simulink model "FAN_FW"  (R2018b)
settings: Solver=ode45  StartTime=0.0  StopTime=40  FixedStep=Ts  RelTol=1e-4  EnableMultiTasking=on
InitFcn:
  | Ts = 1e-4;
  | 
  | Rs = 40;
  | Ld = 0.22;
  | Lq = 0.25;
  | Pn = 4;
  | flux = 0.195;
  | J = 0.000311;
  | 
  | umax = 311/sqrt(3);
  | 
  | kp_cur = Ld*1142;
  | ki_cur = Rs*1142;
  | 
  | 
  | kp_speed = 2*1.7*1*2*pi*J/2;
  | ki_speed = J*(1*2*pi/2)^2;
  | 
  | %kp_speed = 0.0195/5;
  | %ki_speed = 0.0195*50/25;
  | 
  | kp_comp = 0.65;
  | ki_comp = 0.001*pi*kp_comp;
  | 
  | %kp_FW = 0.004;
  | %ki_FW = 0.008;
  | 
  | kp_FW = 0.00004;
  | ki_FW = 0.0004;
  | %kp_FW = 0.00004;
  | %ki_FW = 0.0004;
undefined symbols (not defined in the file or in its folder): DiscIntNeverNeededParam
libraries: powerlib x5, simulink x4
Description:
  | %2020.11.18 98X机型
  | %Rs = 1.415;
  | %Ld = 15.05e-3;
  | %Lq = 18.65e-3;
  | %Pn = 3;
  | %flux = 0.222;
  | %J = 0.000355;
  | %kp_cur = Ld*590.7;
  | %ki_cur = Rs*590.7;
  | %kp_speed = 2*1.7*1*2*pi*J;
  | %ki_speed = J*(1*2*pi)^2;
  | %kp_FW = 0.0001;
  | %ki_FW = 0.00001;
  | 
  | %2020.11.18 海信机型
  | %Rs = 0.8975;
  | %Ld = 15e-3;
  | %Lq = 19e-3;
  | %Pn = 3;
  | %flux = 0.1764;
  | %J = 0.000311;
  | 
  | %2020.11.18 风机机型
  | %Rs = 49.5;
  | %Ld = 0.22;
  | %Lq = 0.25;
  | %Pn = 4;
  | %flux = 0.195;
  | %J = 0.000311;
settings Model: Creator=SUN  LastModifiedBy=liangjin
settings SolverCC: ZeroCrossControl=DisableAll
settings DataIOCC: LimitDataPoints=on  SaveFormat=Array
settings OptimizationCC: ExpressionDepthLimit=2147483647  InitFltsAndDblsToZero=on  LifeSpan=inf
settings DebuggingCC: UnderspecifiedInitializationDetection=Classic  MergeDetectMultiDrivingBlocksExec=none  SolverPrmCheckMsg=warning  FcnCallInpInsideContextMsg=warning  StateNameClashWarn=warning  SFUnexpectedBacktrackingDiag=warning  SFNoUnconditionalDefaultTransitionDiag=warning  SFExecutionAtInitializationDiag=none
settings HardwareCC: ProdBitPerPointer=32  ProdBitPerSizeT=32  ProdBitPerPtrDiffT=32  ProdLargestAtomicFloat=None  ProdIntDivRoundTo=Undefined  ProdEndianess=Unspecified  ProdWordSize=32  ProdHWDeviceType=32-bit Generic
settings ModelReferenceCC: PropagateSignalLabelsOutOfModel=off
settings SFSimCC: SimUseLocalCustomCode=off
settings RTWCC: RTWUseLocalCustomCode=off
settings CodeAppCC: StateflowObjectComments=on
settings GRTTargetCC: TargetLangStandard=C89/C90 (ANSI)  GeneratePreprocessorConditionals=Disable all  CombineOutputUpdateFcns=off  GRTInterface=on
settings ConfigComp: CovMetricSettings=dw  CovHtmlReporting=on  CovSaveCumulativeToWorkspaceVar=on  CovSaveSingleToWorkspaceVar=on  CovExternalEMLEnable=off  CovSFcnEnable=off
settings SimscapeCC: SimscapeNormalizeSystem=off

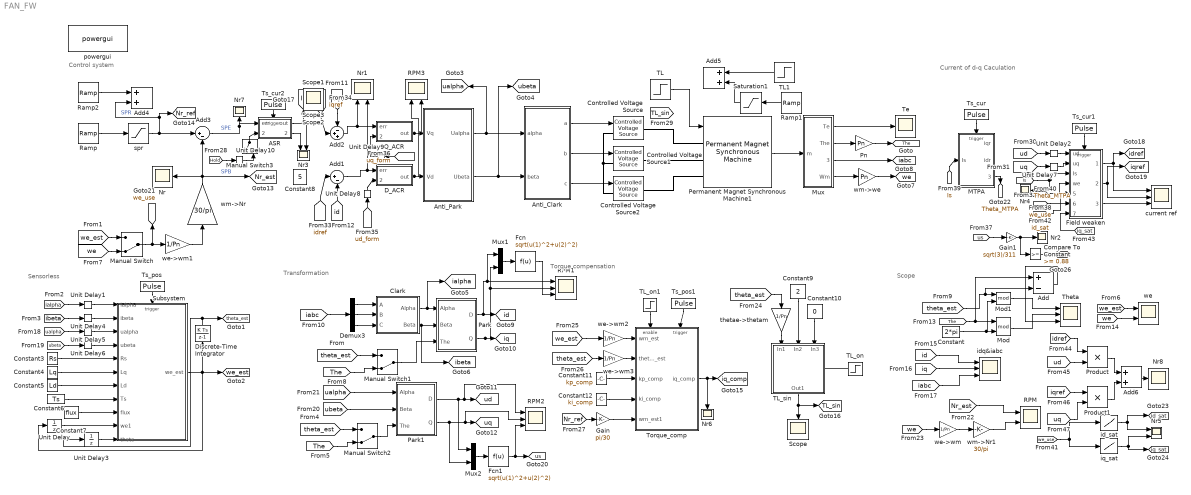
== system FAN_FW ==
  note: Torque compensation
  note: Scope
  note: Control system
  note: Transformation
  note: Sensorless
  note: Current of d-q Caculation
  ASR : Subsystem
  Add : Sum  Inputs=+-
  Add1 : Sum  Inputs=|+-
  Add2 : Sum  Inputs=-++
  Add3 : Sum  Inputs=|+-
  Add4 : Sum
  Add5 : Sum
  Add6 : Sum
  Anti_Clark : Subsystem
  Anti_Park : Subsystem
  Clark : Subsystem
  Compare To Constant : simulink/Logic and Bit Operations/Compare To Constant  relop=>=  const=0.88  OutDataTypeStr=boolean
  Constant : Constant  Value=2*pi
  Constant10 : Constant  Value=0
  Constant11 : Constant  Value=kp_comp
  Constant12 : Constant  Value=ki_comp
  Constant3 : Constant  Value=Rs
  Constant4 : Constant  Value=Lq
  Constant5 : Constant  Value=Ld
  Constant6 : Constant  Value=Ts
  Constant7 : Constant  Value=flux
  Constant8 : Constant  Value=5
  Constant9 : Constant  Value=2  SampleTime=Ts
  Controlled Voltage Source : powerlib/Electrical Sources/Controlled Voltage Source  Initialize=on  Source_Type=AC  Amplitude=0  Phase=0  Frequency=0  Measurements=Voltage
      settings: SourceProductName=Simscape Electrical
  Controlled Voltage Source1 : powerlib/Electrical Sources/Controlled Voltage Source  Initialize=on  Source_Type=AC  Amplitude=0  Phase=0  Frequency=0  Measurements=Voltage
      settings: SourceProductName=Simscape Electrical
  Controlled Voltage Source2 : powerlib/Electrical Sources/Controlled Voltage Source  Initialize=on  Source_Type=AC  Amplitude=0  Phase=0  Frequency=0  Measurements=Voltage
      settings: SourceProductName=Simscape Electrical
  D_ACR : Subsystem
  Demux3 : Demux  Outputs=3
  Discrete-Time Integrator : DiscreteIntegrator  gainval=1  SampleTime=Ts  ICPrevOutput=DiscIntNeverNeededParam  ICPrevScaledInput=DiscIntNeverNeededParam
  Fcn : Fcn  Expr=sqrt(u(1)^2+u(2)^2)
  Fcn1 : Fcn  Expr=sqrt(u(1)^2+u(2)^2)
  Field weaken : Subsystem
  Gain : Gain  Gain=pi/30
  Gain1 : Gain  Gain=sqrt(3)/311
  MTPA : Subsystem
  Manual Switch : ManualSwitch  CurrentSetting=0
  Manual Switch1 : ManualSwitch  CurrentSetting=0
  Manual Switch2 : ManualSwitch  CurrentSetting=0
  Manual Switch3 : ManualSwitch
  Mod : Math  Operator=mod  SaturateOnIntegerOverflow=on
  Mod1 : Math  Operator=mod  SaturateOnIntegerOverflow=on
  Mux : Subsystem
  Mux1 : Mux  Inputs=2
  Mux2 : Mux  Inputs=2
  Nr{,2,4,6..8} (6 alike) : Scope
  Nr1 : Scope  NumInputPorts=2
  Nr3 : Scope  NumInputPorts=2
  Nr5 : Scope  NumInputPorts=2
  Park : Subsystem
  Park1 : Subsystem
  Permanent Magnet Synchronous Machine1 : powerlib/Machines/Permanent Magnet Synchronous Machine  NbPhases=3  FluxDistribution=Sinusoidal  RotorType=Salient-pole  MechanicalLoad=Torque Tm  PresetModel=No  ShowDetailedParameters=on  MeasurementBus=off  Resistance=40  Inductance=8.5e-3  dqInductances=[0.22,0.25]  La=0.000835  MachineConstant=Flux linkage established by magnets (V.s)  Flux=0.195  VoltageCst=141.4764  TorqueCst=1.17  Flat=120  Mechanical=[0.000311 0.0000001 4 0]  PolePairs=3  InitialConditions=[0,0, 0,0]  InitialConditions5ph=[0 0 0 0 0 0]  TsPowergui=0  TsBlock=Ts  RefAngle=Aligned with phase A axis (original Park)
  Pn : Gain  Gain=Pn
  Product : Product
  Product1 : Product
  Q_ACR : Subsystem
  RPM : Scope  NumInputPorts=2
  RPM1 : Scope  NumInputPorts=3
  RPM2 : Scope  NumInputPorts=3
  RPM3 : Scope  NumInputPorts=2
  Ramp : simulink/Sources/Ramp  slope=500  start=0  InitialOutput=0
  Ramp1 : simulink/Sources/Ramp  slope=0.2  start=1  InitialOutput=0
  Ramp2 : simulink/Sources/Ramp  slope=-500  start=18  InitialOutput=0
  Saturation1 : Saturate  UpperLimit=4  LowerLimit=0
  Scope{,1..3} (4 alike) : Scope
  Subsystem : Subsystem
  TL : Step  After=0.8  SampleTime=Ts
  TL1 : Step  Time=15  After=-1  SampleTime=Ts
  TL_on : Step  Time=4  SampleTime=0
  TL_on1 : Step  Time=4  SampleTime=0
  TL_sin : Subsystem
  Te : Scope
  Theta : Scope  NumInputPorts=3
  Torque_comp : Subsystem
  Ts_cur : DiscretePulseGenerator  PulseType=Time based  Period=Ts  PulseWidth=50
  Ts_cur1 : DiscretePulseGenerator  PulseType=Time based  Period=Ts  PulseWidth=50
  Ts_cur2 : DiscretePulseGenerator  PulseType=Time based  Period=Ts  PulseWidth=50
  Ts_pos : DiscretePulseGenerator  PulseType=Time based  Period=Ts  PulseWidth=50
  Ts_pos1 : DiscretePulseGenerator  PulseType=Time based  Period=Ts  PulseWidth=50
  Unit Delay{,1..7} (8 alike) : UnitDelay  SampleTime=Ts
  Unit Delay10 : UnitDelay  SampleTime=-1
  Unit Delay8 : UnitDelay  SampleTime=-1
  Unit Delay9 : UnitDelay  SampleTime=-1
  current ref : Scope  NumInputPorts=3
  id_sat : Lookup_n-D  NumberOfTableDimensions=1  BreakpointsForDimension1=[20:20:4000]  Table=|  InternalRulePriority=Speed  RndMeth=Simplest  InputSameDT=on
      | [0
      | 0
      | 0
      | 0
      | 0
      | 0
      | 0
      | 0
      | 0
      | 0
      | 0
      | 0
      | 0
      | 0
      | 0
      | 0
      | 0
      | 0
      | 0
      | 0
      | 0
      | 0
      | 0
      | 0
      | 0
      | 0
      | 0
      | 0
      | 0
      | 0
      | 0
      | 0
      | 0
      | 0
      | -1.4282156
      | -1.993261291
      | -2.500274735
      | -2.95762852
      | -3.372109996
      | -3.749295371
      | -4.093818374
      | -4.409567747
      | -4.699835339
      | -4.967429105
      | -5.214760613
      | -5.443913731
      | -5.656699168
      | -5.854698247
      | -6.039298363
      | -6.211721953
      | -6.373050352
      | -6.524243572
      | -6.666156819
      | -6.799554349
      | -6.925121177
      | -7.043473009
      | -7.155164714
      | -7.260697576
      | -7.360525538
      | -7.455060585
      | -7.544677419
      | -7.629717516
      | -7.710492675
      | -7.78728811
      | -7.860365185
      | -7.9299638
      | -7.996304512
      | -8.059590407
      | -8.120008759
      | -8.177732505
      | -8.232921567
      | -8.285724019
      | -8.336277143
      | -8.38470837
      | -8.43113613
      | -8.475670606
      | -8.518414431
      | -8.559463299
      | -8.598906531
      | -8.636827584
      | -8.673304508
      | -8.708410367
      | -8.74221362
      | -8.774778469
      | -8.806165173
      | -8.836430342
      | -8.865627195
      | -8.89380581
      | -8.92101334
      | -8.947294219
      | -8.972690352
      | -8.997241281
      | -9.020984353
      | -9.043954856
      | -9.066186163
      | -9.087709851
      | -9.108555817
      | -9.128752388
      | -9.148326416
      | -9.167303371
      | -9.185707429
      | -9.203561544
      | -9.220887527
      | -9.237706113
      | -9.254037024
      | -9.269899028
      | -9.285309992
      | -9.30028694
      | -9.314846093
      | -9.329002919
      | -9.342772173
      | -9.356167938
      | -9.369203658
      | -9.381892176
      | -9.394245766
      | -9.406276161
      | -9.417994582
      | -9.429411766
      | -9.440537991
      | -9.451383096
      | -9.46195651
      | -9.472267265
      | -9.48232402
      | -9.492135081
      | -9.501708414
      | -9.511051664
      | -9.52017217
      | -9.52907698
      | -9.537772864
      | -9.546266329
      | -9.554563629
      | -9.562670776
      | -9.570593555
      | -9.57833753
      | -9.585908059
      | -9.593310297
      | -9.60054921
      | -9.607629581
      | -9.61455602
      | -9.621332968
      | -9.627964709
      | -9.634455372
      | -9.640808941
      | -9.64702926
      | -9.653120038
      | -9.659084857
      | -9.664927176
      | -9.670650332
      | -9.676257554
      | -9.681751959
      | -9.687136559
      | -9.692414269
      | -9.697587906
      | -9.702660194
      | -9.707633768
      | -9.71251118
      | -9.717294898
      | -9.721987311
      | -9.726590734
      | -9.731107406
      | -9.735539499
      | -9.739889116
      | -9.744158294
      | -9.748349008
      | -9.752463174
      | -9.756502648
      | -9.76046923
      | -9.764364667
      | -9.768190654
      | -9.771948834
      | -9.775640804
      | -9.779268112
      | -9.782832262
      | -9.786334715
      | -9.789776889
      | -9.793160162
      | -9.796485872
      | -9.799755319
      | -9.802969768
      | -9.806130448
      | -9.809238552
      | -9.812295243
      | -9.81530165
      | -9.818258872
      | -9.821167977
      | -9.824030004
      | -9.826845967
      | -9.82961685
      | -9.83234361
      | -9.835027183
      | -9.837668475
      | -9.840268372
      | -9.842827735
      | -9.845347404
      | -9.847828197
      | -9.850270911
      | -9.852676321
      | -9.855045185
      | -9.85737824
      | -9.859676205
      | ]
  idq&iabc : Scope  NumInputPorts=3
  iq_sat : Lookup_n-D  NumberOfTableDimensions=1  BreakpointsForDimension1=[20:20:4000]  Table=|  InternalRulePriority=Speed  RndMeth=Simplest  InputSameDT=on
      | [10
      | 10
      | 10
      | 10
      | 10
      | 10
      | 10
      | 10
      | 10
      | 10
      | 10
      | 10
      | 10
      | 10
      | 10
      | 10
      | 10
      | 10
      | 10
      | 10
      | 10
      | 10
      | 10
      | 10
      | 10
      | 10
      | 10
      | 10
      | 10
      | 10
      | 10
      | 10
      | 10
      | 10
      | 9.897484539
      | 9.799332091
      | 9.682387425
      | 9.552613964
      | 9.414290955
      | 9.270533114
      | 9.123631465
      | 8.97528341
      | 8.826751825
      | 8.678977364
      | 8.532659125
      | 8.388313495
      | 8.246317634
      | 8.10694199
      | 7.970374852
      | 7.836741056
      | 7.706116351
      | 7.578538501
      | 7.454015915
      | 7.332534395
      | 7.214062426
      | 7.098555344
      | 6.985958625
      | 6.87621049
      | 6.769243961
      | 6.664988498
      | 6.563371287
      | 6.464318264
      | 6.36775492
      | 6.273606928
      | 6.18180064
      | 6.092263465
      | 6.004924158
      | 5.919713039
      | 5.836562153
      | 5.755405379
      | 5.67617851
      | 5.598819294
      | 5.523267457
      | 5.449464703
      | 5.377354699
      | 5.306883056
      | 5.237997288
      | 5.170646772
      | 5.104782705
      | 5.040358051
      | 4.977327487
      | 4.915647352
      | 4.855275587
      | 4.796171685
      | 4.738296629
      | 4.681612844
      | 4.626084136
      | 4.571675646
      | 4.518353792
      | 4.466086223
      | 4.41484177
      | 4.364590396
      | 4.315303153
      | 4.266952139
      | 4.219510452
      | 4.172952153
      | 4.127252226
      | 4.082386538
      | 4.038331808
      | 3.995065568
      | 3.952566132
      | 3.910812564
      | 3.869784647
      | 3.829462856
      | 3.789828327
      | 3.750862836
      | 3.712548767
      | 3.674869091
      | 3.637807343
      | 3.6013476
      | 3.565474459
      | 3.530173016
      | 3.495428846
      | 3.461227989
      | 3.427556926
      | 3.394402566
      | 3.36175223
      | 3.329593631
      | 3.297914864
      | 3.266704389
      | 3.23595102
      | 3.205643908
      | 3.175772532
      | 3.146326683
      | 3.117296459
      | 3.088672246
      | 3.060444715
      | 3.032604806
      | 3.005143721
      | 2.978052915
      | 2.951324087
      | 2.924949168
      | 2.898920319
      | 2.873229917
      | 2.847870553
      | 2.822835019
      | 2.798116307
      | 2.773707596
      | 2.749602251
      | 2.725793813
      | 2.702275997
      | 2.679042682
      | 2.656087907
      | 2.633405868
      | 2.61099091
      | 2.588837522
      | 2.566940337
      | 2.545294119
      | 2.523893767
      | 2.502734308
      | 2.481810888
      | 2.461118776
      | 2.440653356
      | 2.420410124
      | 2.400384682
      | 2.380572741
      | 2.360970112
      | 2.341572703
      | 2.32237652
      | 2.303377661
      | 2.284572314
      | 2.265956753
      | 2.24752734
      | 2.229280514
      | 2.211212798
      | 2.193320789
      | 2.175601161
      | 2.158050659
      | 2.1406661
      | 2.123444368
      | 2.106382414
      | 2.089477254
      | 2.072725965
      | 2.056125686
      | 2.039673615
      | 2.023367006
      | 2.00720317
      | 1.991179471
      | 1.975293326
      | 1.959542202
      | 1.943923615
      | 1.928435132
      | 1.913074362
      | 1.897838962
      | 1.882726634
      | 1.867735119
      | 1.852862202
      | 1.838105707
      | 1.823463498
      | 1.808933475
      | 1.794513578
      | 1.780201779
      | 1.765996087
      | 1.751894542
      | 1.73789522
      | 1.723996225
      | 1.710195695
      | 1.696491794
      | 1.682882717
      | 1.669366687
      | ]
  powergui : powerlib/powergui  SimulationMode=Discrete  SampleTime=1e-5  frequency=60  Iterations=50  frequencyindice=0  Pbase=100e6  ErrMax=1e-4  UnitsV=kV  UnitsW=MW  buscounter=0  FunctionMessages=off  echomessages=off  EnableUseOfTLC=off  CurrentSourceSwitches=off  DisableSnubberDevices=off  DisableRonSwitches=off  DisableVfSwitches=off  DisplayEquations=off  SolverType=Tustin/Backward Euler (TBE)  Interpol=off  ExternalGateDelay=off  methode=off  Ts=100  x0status=blocks  SPID=off  SwTol=0  HookPort=off  RestoreLinks=warning  ResistiveCurrentMeasurement=off  Frange=[0:2:500]  Ylog=off  Xlog=on  ShowGrid=off  save=off  variable=ZData  structure=0  ZoomFFT=on  StartTime=0.0  cycles=1  DisplayStyle=1  fundamental=60  FreqAxis=off  MaxFrequency=1000  frequencyindicesteady=1  RmsSteady=1  display=off
  spr : Saturate  UpperLimit=8000  LowerLimit=-1000
  thetae->thetam : Gain  Gain=1/Pn
  we : Scope  NumInputPorts=2
  we->wm{,1..3} (4 alike) : Gain  Gain=1/Pn
  wm->Nr : Gain  Gain=30/pi
  wm->Nr1 : Gain  Gain=30/pi
  wm->we : Gain  Gain=Pn
  tag scope: Hold=global, Is=global, Nr_est=global, Nr_ref=global, TL_sin=global, The=global, Theta_MTPA=global, iabc=global, ialpha=global, ibeta=global, id=global, id_sat=global, idref=global, iq=global, iq_comp=global, iq_sat=global, iqref=global, theta_est=global, ualpha=global, ubeta=global, ud=global, uq=global, us=global, we=global, we_est=global, we_use=global
  wires:
  Permanent Magnet Synchronous Machine1/1 -> Mux/1(m)
  Add3/1 -> ASR/1(err), Nr7/1  "SPE"
  wm->Nr/1 -> [Nr_est], Add3/2, Nr/1  "SPB"
  Mux/1(Te) -> Te/1
  Mux/2(The) -> Pn/1
  Pn/1 -> [The]
  Mux/4(Wm) -> wm->we/1
  Mux/3(Iabc) -> [iabc]
  Clark/1(Alpha) -> [ialpha], Park/1(Alpha)
  Demux3/1 -> Clark/1(A)
  Demux3/2 -> Clark/2(B)
  Demux3/3 -> Clark/3(C)
  Clark/2(Beta) -> Park/2(Beta), [ibeta]
  Q_ACR/1(out) -> RPM3/2, Anti_Park/1(Vq)
  D_ACR/1(out) -> RPM3/1, Anti_Park/2(Vd)
  Anti_Clark/2(b) -> Controlled Voltage Source1/1
  Anti_Clark/3(c) -> Controlled Voltage Source2/1
  Constant/1 -> Mod1/2, Mod/2
  Mod/1 -> Theta/2
  wm->we/1 -> [we]
  Ramp/1 -> spr/1
  we->wm1/1 -> wm->Nr/1
  [we_est] -> we/1
  [we_est] -> Manual Switch/1
  [we] -> Manual Switch/2
  [theta_est] -> Manual Switch1/1
  Manual Switch1/1 -> Park/3(The)
  [The] -> Manual Switch1/2
  Park/1(D) -> Mux1/1, RPM1/1, [id]
  Park/2(Q) -> Mux1/2, RPM1/2, [iq]
  [The] -> Add/1, Mod/1
  [id] -> idq&iabc/1
  [iq] -> idq&iabc/2
  [iabc] -> idq&iabc/3
  [id] -> Add1/2
  [iq] -> Add2/1
  Manual Switch/1 -> we->wm1/1, [we_use]
  [The] -> Manual Switch2/2
  Manual Switch2/1 -> Park1/3(The)
  [theta_est] -> Manual Switch2/1
  [ubeta] -> Park1/2(Beta)
  [ualpha] -> Park1/1(Alpha)
  Park1/1(D) -> Mux2/1, [ud], RPM2/1
  Park1/2(Q) -> Mux2/2, RPM2/2, [uq]
  Anti_Park/1(Ualpha) -> [ualpha], Anti_Clark/1(alpha)
  Anti_Park/2(Ubeta) -> [ubeta], Anti_Clark/2(beta)
  Subsystem/1(we_est) -> Discrete-Time Integrator/1, [we_est], Unit Delay/1
  Constant3/1 -> Subsystem/5(Rs)
  Constant4/1 -> Subsystem/6(Lq)
  Constant5/1 -> Subsystem/7(Ld)
  Constant6/1 -> Subsystem/8(Ts)
  Constant7/1 -> Subsystem/9(flux)
  Unit Delay/1 -> Subsystem/10(we1)
  Ts_pos/1 -> Subsystem/Trigger
  Unit Delay3/1 -> Subsystem/11(theta)
  [theta_est] -> Add/2, Mod1/1
  Mod1/1 -> Theta/1
  [iabc] -> Demux3/1
  Discrete-Time Integrator/1 -> [theta_est], Unit Delay3/1
  Anti_Clark/1(a) -> Controlled Voltage Source/1
  [ialpha] -> Unit Delay1/1
  [ibeta] -> Unit Delay4/1
  [ualpha] -> Unit Delay5/1
  [ubeta] -> Unit Delay6/1
  [we] -> we->wm/1
  we->wm/1 -> wm->Nr1/1
  wm->Nr1/1 -> RPM/2
  [Nr_est] -> RPM/1
  spr/1 -> [Nr_ref], Add4/2, Add3/1  "SPR"
  Ts_cur/1 -> MTPA/Trigger
  [we] -> we/2
  [theta_est] -> thetae->thetam/1
  thetae->thetam/1 -> TL_sin/1(In1)
  Constant9/1 -> TL_sin/2(In2)
  Constant10/1 -> TL_sin/3(In3)
  TL_on/1 -> TL_sin/Enable
  TL_sin/1(Out1) -> [TL_sin], Scope/1
  we->wm2/1 -> Torque_comp/1(wm_est)
  we->wm3/1 -> Torque_comp/2(thetam_est)
  Constant11/1 -> Torque_comp/3(kp_comp)
  Constant12/1 -> Torque_comp/4(ki_comp)
  Torque_comp/1(iq_comp) -> Nr6/1, [iq_comp]
  [Nr_ref] -> Gain/1
  Gain/1 -> Torque_comp/5(wm_est1)
  Ts_pos1/1 -> Torque_comp/Trigger
  TL_on1/1 -> Torque_comp/Enable
  [we_est] -> we->wm2/1
  [theta_est] -> we->wm3/1
  [ud] -> Unit Delay2/1
  [uq] -> Unit Delay7/1
  [Is] -> Nr4/1, Field weaken/3(Is)
  Ts_cur1/1 -> Field weaken/Trigger
  Field weaken/1(idref) -> current ref/1, [idref]
  Field weaken/2(iqref) -> [iqref], current ref/2
  Add/1 -> Theta/3
  Mux1/1 -> Fcn/1
  Field weaken/3(jiaodu) -> current ref/3
  Mux2/1 -> Fcn1/1
  Fcn1/1 -> [us], RPM2/3
  Unit Delay1/1 -> Subsystem/1(ialpha)
  Unit Delay4/1 -> Subsystem/2(ibeta)
  Unit Delay5/1 -> Subsystem/3(ualpha)
  Unit Delay6/1 -> Subsystem/4(ubeta)
  Unit Delay2/1 -> Field weaken/1(ud)
  Unit Delay7/1 -> Field weaken/2(uq)
  [ud_form] -> Unit Delay8/1
  Unit Delay8/1 -> D_ACR/2(ud_form)
  [uq_form] -> Unit Delay9/1
  Unit Delay9/1 -> Q_ACR/2(uq_form)
  [us] -> Gain1/1
  Gain1/1 -> Compare To Constant/1, Nr2/1
  [we_use] -> Field weaken/4(we)
  Ramp1/1 -> Saturation1/1
  Ramp2/1 -> Add4/1
  TL1/1 -> Add5/1
  [Is] -> MTPA/1(Is)
  MTPA/3(Theta_MTPA) -> [Theta_MTPA]
  [Theta_MTPA] -> Field weaken/5(Theta_MTPA)
  [we_use] -> id_sat/1, iq_sat/1
  id_sat/1 -> Nr5/1, [id_sat]
  iq_sat/1 -> [iq_sat], Nr5/2
  [id_sat] -> Field weaken/6(id_sat)
  [iq_sat] -> Field weaken/7(iq_sat)
  Add1/1 -> Nr1/2, D_ACR/1(err)
  Add2/1 -> Nr1/1, Q_ACR/1(err)
  ASR/1(out) -> Nr3/2, [Is]
  ASR/2(speed_sat) -> Nr3/1
  Compare To Constant/1 -> [Hold]
  [Hold] -> Unit Delay10/1
  Manual Switch3/1 -> ASR/2(Hold)
  Unit Delay10/1 -> Manual Switch3/2
  [idref] -> Product/1
  [ud] -> Product/2
  [iqref] -> Product1/1
  [uq] -> Product1/2
  Product/1 -> Add6/1
  Product1/1 -> Add6/2
  Add6/1 -> Nr8/1
  [idref] -> Add1/1
  [iqref] -> Add2/2
  Ts_cur2/1 -> ASR/Trigger
  Fcn/1 -> RPM1/3
  Saturation1/1 -> Add5/2
  TL/1 -> Permanent Magnet Synchronous Machine1/1
  connections:
  Controlled Voltage Source/LConn1 -- Controlled Voltage Source2/LConn1 -- Controlled Voltage Source1/LConn1
  Controlled Voltage Source/RConn1 -- Permanent Magnet Synchronous Machine1/LConn1
  Controlled Voltage Source1/RConn1 -- Permanent Magnet Synchronous Machine1/LConn2
  Controlled Voltage Source2/RConn1 -- Permanent Magnet Synchronous Machine1/LConn3

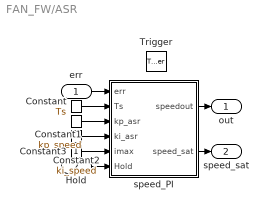
== system FAN_FW/ASR ==
  err : Inport
  Hold : Inport  Port=2
  Trigger : TriggerPort  VariantControl=Variant  PortDimensions=1
  Constant : Constant  Value=Ts
  Constant1 : Constant  Value=kp_speed
  Constant2 : Constant  Value=ki_speed
  Constant3 : Constant
  speed_PI : MATLAB Function  TreatAsAtomicUnit=on
  out : Outport
  speed_sat : Outport  Port=2
  wires:
  speed_PI/1(speedout) -> out/1
  speed_PI/2(speed_sat) -> speed_sat/1
  Hold/1 -> speed_PI/6(Hold)
  Constant2/1 -> speed_PI/4(ki_asr)
  Constant3/1 -> speed_PI/5(imax)
  Constant/1 -> speed_PI/2(Ts)
  err/1 -> speed_PI/1(err)
  Constant1/1 -> speed_PI/3(kp_asr)

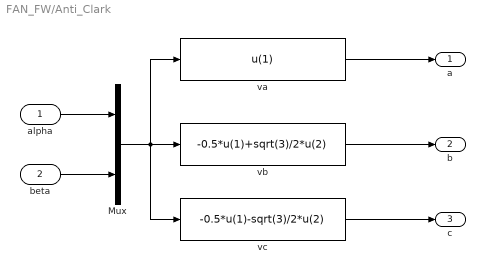
== system FAN_FW/Anti_Clark ==
  alpha : Inport
  beta : Inport  Port=2
  Mux : Mux  Inputs=2
  va : Fcn  Expr=u(1)
  vb : Fcn  Expr=-0.5*u(1)+sqrt(3)/2*u(2)
  vc : Fcn  Expr=-0.5*u(1)-sqrt(3)/2*u(2)
  a : Outport
  b : Outport  Port=2
  c : Outport  Port=3
  wires:
  va/1 -> a/1
  beta/1 -> Mux/2
  alpha/1 -> Mux/1
  Mux/1 -> vc/1, vb/1, va/1
  vb/1 -> b/1
  vc/1 -> c/1

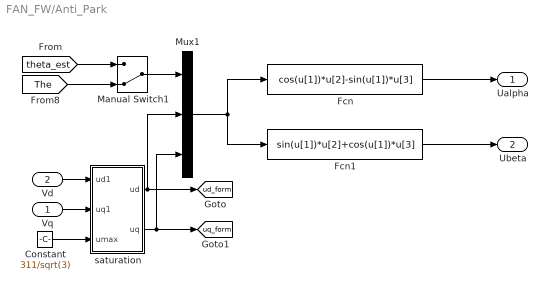
== system FAN_FW/Anti_Park ==
  Vq : Inport
  Vd : Inport  Port=2
  Constant : Constant  Value=311/sqrt(3)
  Fcn : Fcn  Expr=cos(u[1])*u[2]-sin(u[1])*u[3]
  Fcn1 : Fcn  Expr=sin(u[1])*u[2]+cos(u[1])*u[3]
  Manual Switch1 : ManualSwitch  CurrentSetting=0
  Mux1 : Mux  Inputs=3
  saturation : MATLAB Function  TreatAsAtomicUnit=on
  Ualpha : Outport
  Ubeta : Outport  Port=2
  tag scope: ud_form=global, uq_form=global
  wires:
  Fcn1/1 -> Ubeta/1
  Fcn/1 -> Ualpha/1
  Mux1/1 -> Fcn/1, Fcn1/1
  Manual Switch1/1 -> Mux1/1
  [The] -> Manual Switch1/2
  [theta_est] -> Manual Switch1/1
  Vd/1 -> saturation/1(ud1)
  Vq/1 -> saturation/2(uq1)
  saturation/1(ud) -> Mux1/2, [ud_form]
  saturation/2(uq) -> [uq_form], Mux1/3
  Constant/1 -> saturation/3(umax)

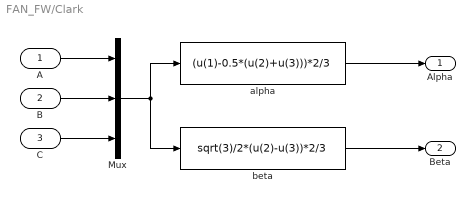
== system FAN_FW/Clark ==
  A : Inport
  B : Inport  Port=2
  C : Inport  Port=3
  Mux : Mux  Inputs=3
  alpha : Fcn  Expr=(u(1)-0.5*(u(2)+u(3)))*2/3
  beta : Fcn  Expr=sqrt(3)/2*(u(2)-u(3))*2/3
  Alpha : Outport
  Beta : Outport  Port=2
  wires:
  alpha/1 -> Alpha/1
  B/1 -> Mux/2
  C/1 -> Mux/3
  A/1 -> Mux/1
  Mux/1 -> beta/1, alpha/1
  beta/1 -> Beta/1

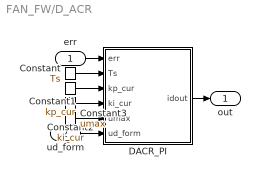
== system FAN_FW/D_ACR ==
  err : Inport
  ud_form : Inport  Port=2
  Constant : Constant  Value=Ts
  Constant1 : Constant  Value=kp_cur
  Constant2 : Constant  Value=ki_cur
  Constant3 : Constant  Value=umax
  DACR_PI : MATLAB Function  TreatAsAtomicUnit=on
  out : Outport
  wires:
  err/1 -> DACR_PI/1(err)
  Constant3/1 -> DACR_PI/5(umax)
  Constant2/1 -> DACR_PI/4(ki_cur)
  Constant/1 -> DACR_PI/2(Ts)
  Constant1/1 -> DACR_PI/3(kp_cur)
  ud_form/1 -> DACR_PI/6(ud_form)
  DACR_PI/1(idout) -> out/1

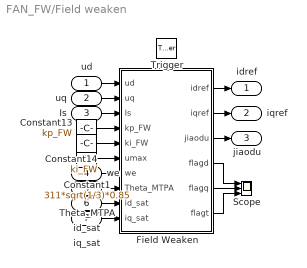
== system FAN_FW/Field weaken ==
  ud : Inport
  uq : Inport  Port=2
  Is : Inport  Port=3
  we : Inport  Port=4
  Theta_MTPA : Inport  Port=5
  id_sat : Inport  Port=6
  iq_sat : Inport  Port=7
  Trigger : TriggerPort  VariantControl=Variant  PortDimensions=1
  Constant1 : Constant  Value=311*sqrt(1/3)*0.85
  Constant13 : Constant  Value=kp_FW
  Constant14 : Constant  Value=ki_FW
  Field Weaken : MATLAB Function  TreatAsAtomicUnit=on
  Scope : Scope  NumInputPorts=3
  idref : Outport
  iqref : Outport  Port=2
  jiaodu : Outport  Port=3
  wires:
  Constant13/1 -> Field Weaken/4(kp_FW)
  Field Weaken/1(idref) -> idref/1
  Constant14/1 -> Field Weaken/5(ki_FW)
  uq/1 -> Field Weaken/2(uq)
  Constant1/1 -> Field Weaken/6(umax)
  Field Weaken/2(iqref) -> iqref/1
  ud/1 -> Field Weaken/1(ud)
  Is/1 -> Field Weaken/3(Is)
  Field Weaken/3(jiaodu) -> jiaodu/1
  we/1 -> Field Weaken/7(we)
  Theta_MTPA/1 -> Field Weaken/8(Theta_MTPA)
  Field Weaken/4(flagd) -> Scope/1
  Field Weaken/5(flagq) -> Scope/2
  Field Weaken/6(flagt) -> Scope/3
  id_sat/1 -> Field Weaken/9(id_sat)
  iq_sat/1 -> Field Weaken/10(iq_sat)

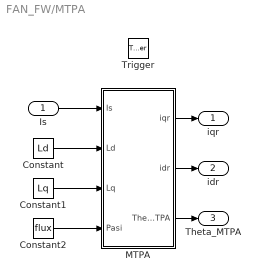
== system FAN_FW/MTPA ==
  Is : Inport
  Trigger : TriggerPort  VariantControl=Variant  PortDimensions=1
  Constant : Constant  Value=Ld
  Constant1 : Constant  Value=Lq
  Constant2 : Constant  Value=flux
  MTPA : MATLAB Function  TreatAsAtomicUnit=on
  iqr : Outport
  idr : Outport  Port=2
  Theta_MTPA : Outport  Port=3
  wires:
  MTPA/1(iqr) -> iqr/1
  Is/1 -> MTPA/1(Is)
  Constant/1 -> MTPA/2(Ld)
  Constant1/1 -> MTPA/3(Lq)
  Constant2/1 -> MTPA/4(Pasi)
  MTPA/2(idr) -> idr/1
  MTPA/3(Theta_MTPA) -> Theta_MTPA/1

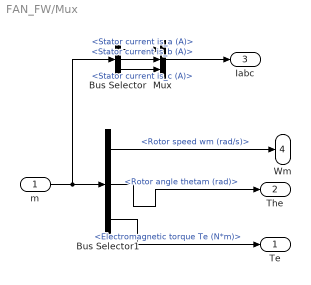
== system FAN_FW/Mux ==
  m : Inport
  Bus Selector : BusSelector  OutputSignals=Stator current is_a (A),Stator current is_b (A),Stator current is_c (A)
  Bus Selector1 : BusSelector  OutputSignals=Rotor speed wm (rad/s),Rotor angle thetam (rad),Electromagnetic torque Te (N*m)
  Mux : Mux  Inputs=3
  Te : Outport
  The : Outport  Port=2
  Iabc : Outport  Port=3
  Wm : Outport  Port=4
  wires:
  Bus Selector1/1 -> Wm/1  "<Rotor speed wm (rad/s)>"
  Bus Selector1/2 -> The/1  "<Rotor angle thetam (rad)>"
  Bus Selector1/3 -> Te/1  "<Electromagnetic torque Te (N*m)>"
  m/1 -> Bus Selector/1, Bus Selector1/1
  Bus Selector/2 -> Mux/2  "<Stator current is_b (A)>"
  Bus Selector/3 -> Mux/3  "<Stator current is_c (A)>"
  Bus Selector/1 -> Mux/1  "<Stator current is_a (A)>"
  Mux/1 -> Iabc/1

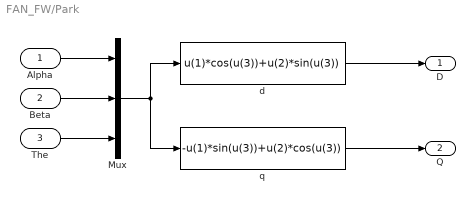
== system FAN_FW/Park ==
  Alpha : Inport
  Beta : Inport  Port=2
  The : Inport  Port=3
  Mux : Mux  Inputs=3
  d : Fcn  Expr=u(1)*cos(u(3))+u(2)*sin(u(3))
  q : Fcn  Expr=-u(1)*sin(u(3))+u(2)*cos(u(3))
  D : Outport
  Q : Outport  Port=2
  wires:
  d/1 -> D/1
  Beta/1 -> Mux/2
  Alpha/1 -> Mux/1
  Mux/1 -> q/1, d/1
  q/1 -> Q/1
  The/1 -> Mux/3

== system FAN_FW/Park1 ==
  Alpha : Inport
  Beta : Inport  Port=2
  The : Inport  Port=3
  Mux : Mux  Inputs=3
  d : Fcn  Expr=u(1)*cos(u(3))+u(2)*sin(u(3))
  q : Fcn  Expr=-u(1)*sin(u(3))+u(2)*cos(u(3))
  D : Outport
  Q : Outport  Port=2
  wires:
  d/1 -> D/1
  Beta/1 -> Mux/2
  Alpha/1 -> Mux/1
  Mux/1 -> q/1, d/1
  q/1 -> Q/1
  The/1 -> Mux/3

== system FAN_FW/Q_ACR ==
  err : Inport
  uq_form : Inport  Port=2
  Constant : Constant  Value=Ts
  Constant1 : Constant  Value=kp_cur
  Constant2 : Constant  Value=ki_cur
  Constant3 : Constant  Value=umax
  QACR_PI : MATLAB Function  TreatAsAtomicUnit=on
  out : Outport
  wires:
  err/1 -> QACR_PI/1(err)
  Constant3/1 -> QACR_PI/5(umax)
  Constant2/1 -> QACR_PI/4(ki_cur)
  Constant/1 -> QACR_PI/2(Ts)
  Constant1/1 -> QACR_PI/3(kp_cur)
  uq_form/1 -> QACR_PI/6(ud_form)
  QACR_PI/1(iqout) -> out/1

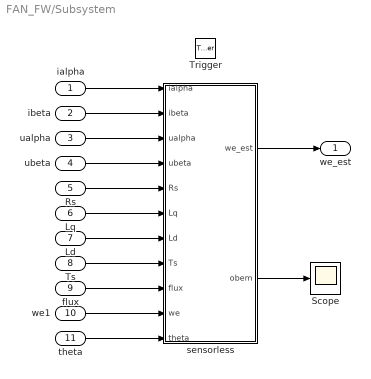
== system FAN_FW/Subsystem ==
  ialpha : Inport
  ibeta : Inport  Port=2
  ualpha : Inport  Port=3
  ubeta : Inport  Port=4
  Rs : Inport  Port=5
  Lq : Inport  Port=6
  Ld : Inport  Port=7
  Ts : Inport  Port=8
  flux : Inport  Port=9
  we1 : Inport  Port=10
  theta : Inport  Port=11
  Trigger : TriggerPort  VariantControl=Variant  PortDimensions=1
  Scope : Scope
  sensorless : MATLAB Function  TreatAsAtomicUnit=on
  we_est : Outport
  wires:
  ualpha/1 -> sensorless/3(ualpha)
  Ts/1 -> sensorless/8(Ts)
  flux/1 -> sensorless/9(flux)
  ialpha/1 -> sensorless/1(ialpha)
  sensorless/1(we_est) -> we_est/1
  Lq/1 -> sensorless/6(Lq)
  ubeta/1 -> sensorless/4(ubeta)
  ibeta/1 -> sensorless/2(ibeta)
  Rs/1 -> sensorless/5(Rs)
  Ld/1 -> sensorless/7(Ld)
  we1/1 -> sensorless/10(we)
  theta/1 -> sensorless/11(theta)
  sensorless/2(obem) -> Scope/1

== system FAN_FW/TL_sin ==
  In1 : Inport
  In2 : Inport  Port=2
  In3 : Inport  Port=3
  Enable : EnablePort
  MATLAB Function : MATLAB Function  TreatAsAtomicUnit=on
  Out1 : Outport
  wires:
  In1/1 -> MATLAB Function/1(Theta_m)
  MATLAB Function/1(TL) -> Out1/1
  In3/1 -> MATLAB Function/3(Theta0)
  In2/1 -> MATLAB Function/2(Amp)

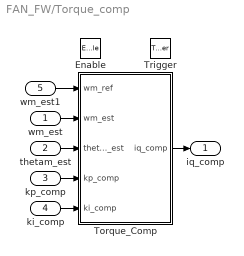
== system FAN_FW/Torque_comp ==
  wm_est : Inport
  thetam_est : Inport  Port=2
  kp_comp : Inport  Port=3
  ki_comp : Inport  Port=4
  wm_est1 : Inport  Port=5
  Enable : EnablePort
  Trigger : TriggerPort  VariantControl=Variant  PortDimensions=1
  Torque_Comp : MATLAB Function  TreatAsAtomicUnit=on
  iq_comp : Outport
  wires:
  Torque_Comp/1(iq_comp) -> iq_comp/1
  kp_comp/1 -> Torque_Comp/4(kp_comp)
  wm_est/1 -> Torque_Comp/2(wm_est)
  ki_comp/1 -> Torque_Comp/5(ki_comp)
  wm_est1/1 -> Torque_Comp/1(wm_ref)
  thetam_est/1 -> Torque_Comp/3(thetam_est)

== matlab function FAN_FW/MTPA/MTPA ==
  data: iqr output; Is input; idr output; Ld input; Lq input; Pasi input; Theta_MTPA output
function [iqr,idr,Theta_MTPA] = MTPA(Is,Ld,Lq,Pasi)

persistent id1 iq1;

if isempty(id1)
    id1=0;iq1=0;
end

iq1 = Is;
id1 = iq1*iq1*(Ld-Lq)/Pasi;

Theta_MTPA = atan(id1/iq1);
idr = id1;
iqr = iq1;

== matlab function FAN_FW/Subsystem/sensorless ==
  data: ialpha input; we_est output; ibeta input; ualpha input; ubeta input; Rs input; Lq input; Ld input; Ts input; flux input; we input; theta input; obem output

function [we_est, obem]  = sensorless(ialpha,ibeta,ualpha,ubeta,Rs,Lq,Ld,Ts,flux,we,theta)

persistent id2 iq2 delta_id delta_iq bemf we1 flag;

if isempty(id2)
    id2=0;iq2=0;delta_id=0;delta_iq=0;bemf=0;we1=0;flag=0;obem=0;
end

ud= cos(theta)*ualpha+sin(theta)*ubeta;
uq=-sin(theta)*ualpha+cos(theta)*ubeta;
id1= cos(theta)*ialpha+sin(theta)*ibeta;
iq1=-sin(theta)*ialpha+cos(theta)*ibeta;

if(bemf < 0)
    flag = 1;
end

we1 = we1+0.715*(we-we1);
temp1 = ud-id2*Rs;
temp1 = temp1+we1*Lq*iq2;
temp1 = temp1*Ts/Ld + id2;
delta_id = delta_id+0.125*((temp1-id1)-delta_id);

temp2 = uq-iq2*Rs;
temp2 = temp2-we1*Ld*id2;
temp2 = temp2-bemf;
temp2 = Ts*temp2/Lq+iq2;
delta_iq = delta_iq+0.5*((temp2-iq1)-delta_iq);

bemf = bemf+delta_iq*Lq/Ts;
if(flag)
    we_est = (bemf+delta_id*Ld/Ts)/flux;
else
    we_est = (bemf-delta_id*Ld/Ts)/flux;
end

obem = bemf;
id2 = id1;
iq2 = iq1;

== matlab function FAN_FW/TL_sin/MATLAB Function ==
  data: Theta_m input; TL output; Amp input; Theta0 input
function TL = fcn(Theta_m,Amp,Theta0)
if isempty(Theta_m)
    Theta_m=0;Amp=0;Theta0=0;TL=0;
end
TL = Amp*sin(Theta_m+Theta0);

== matlab function FAN_FW/Torque_comp/Torque_Comp ==
  data: wm_ref input; iq_comp output; wm_est input; thetam_est input; kp_comp input; ki_comp input
function iq_comp = Torque_Comp(wm_ref,wm_est,thetam_est,kp_comp,ki_comp)

persistent Te temp1 temp2 up ui1 ui2 out1 out2 comp1_fbk comp2_fbk comp1_ref comp2_ref;

if isempty(temp1)
    Te=0; temp1=0; temp2=0; up=0; ui1=0; ui2=0; out1=0; out2=0; iq_comp=0; 
    comp1_fbk=0; comp2_fbk=0; comp1_ref=0; comp2_ref=0;
end

%calc comp sin value
Te = wm_ref-wm_est;
temp1 = Te*sin(thetam_est);
comp1_fbk = 0;
if (wm_ref < 10)
    comp1_ref = 0;
else
    comp1_ref = temp1;
end
up = comp1_ref - comp1_fbk;
ui1 = ui1 + ki_comp*up;
out1 = kp_comp*up + ui1;

%calc comp cos value
temp2 = Te*cos(thetam_est);
comp2_fbk = 0;
if (wm_ref < 10)
    comp2_ref = 0;
else
    comp2_ref = temp2;
end
up = comp2_ref - comp2_fbk;
ui2 = ui2 + ki_comp*up;
out2 = kp_comp*up + ui2;

iq_comp = out1*sin(thetam_est) + out2*cos(thetam_est);

if (iq_comp > 10)
    iq_comp = 10;
elseif (iq_comp < -10)
    iq_comp = -10;
end

== matlab function FAN_FW/Field weaken/Field Weaken ==
  data: idref output; iqref output; ud input; uq input; Is input; kp_FW input; ki_FW input; umax input; jiaodu output; we input; Theta_MTPA input; flagd output; flagq output; flagt output; id_sat input; iq_sat input
function [idref,iqref,jiaodu,flagd,flagq,flagt] = Fieldweaken(ud,uq,Is,kp_FW,ki_FW,umax,we,Theta_MTPA,id_sat,iq_sat)

persistent us gama uout ui temp id1 iq1 gama_sat upper flag_temp1 flag_temp2 flag_temp3 ;

if isempty(us)
    us=0;gama=0;ui=0;temp=0;uout=0;id1=0;iq1=0;gama_sat=0;upper=0;flag_temp1=0;flag_temp2=0;flag_temp3=0;
%     id_sat=0;iq_sat=0;
end
% 
% id_sat = (5.385-0.01537*we+0.000004*we*we);
% iq_sat = (16.82-0.01108*we+0.000002*we*we);
% id_sat = (9.3451-0.0243*we+0.00001*we*we-2*10^(-9)*we*we*we);
% iq_sat = (15.36-0.0085*we+0.000002*we*we);


%gama_sat = k1*asin(id_sat/10);

flag_temp2 = 0;
flag_temp3 = 0;
us = sqrt(ud.^2+uq.^2);
temp = umax - us;

if(temp>0)
    upper = Theta_MTPA;
else
    upper = 0;
end
% 
% if((temp<10)  && (temp>0))
%     uout = gama;
%     temp = 0;
% else
    if(gama == uout)
        ui = ui+temp*ki_FW;
    end
    uout = kp_FW*temp+ui;
% end

% if (uout<=gama_sat)
% %     uout = gama_sat;
%     flag_temp3=1;
% if (uout<=-pi/2)
%     gama = -pi/2;
if (uout<=-0.83)
    gama = -0.83;
    flag_temp3=1;
elseif (uout>=upper)
    gama = upper;
    ui = upper;
else
    gama = uout;
end
    
iq1 = Is*cos(gama);
id1 = Is*sin(gama);
flag_temp1 = 0;

if(id1<id_sat)
%     id1=id_sat;
    flag_temp1 = 1;
end

if(iq1>iq_sat)
    iq1=iq_sat;
    flag_temp2=1;
end

if(id1>0)
    id1=0;
end

if(iq1<-iq_sat)
    iq1=-iq_sat;
end

flagd = flag_temp1;
flagq = flag_temp2;
flagt = flag_temp3;
idref = id1;
iqref = iq1;
jiaodu =rad2deg(gama);

== matlab function FAN_FW/Anti_Park/saturation ==
  data: ud1 input; ud output; uq1 input; umax input; uq output
function [ud,uq] = saturation(ud1,uq1,umax)

persistent us ud2 uq2;

if isempty(us)
    us=0;ud2=0;uq2=0;
end

us = sqrt(ud1.^2+uq1.^2);

if(us>=umax)
    ud2 = ud1*umax/us;
    uq2 = uq1*umax/us;
%     uq2 = sqrt((umax).^2-ud1.^2);
%     ud2 = ud1;
else
    ud2 = ud1;
    uq2 = uq1;
end
    
ud = ud2;
uq = uq2;

== matlab function FAN_FW/Q_ACR/QACR_PI ==
  data: err input; iqout output; Ts input; kp_cur input; ki_cur input; umax input; ud_form input
function iqout  = QACR_PI(err,Ts,kp_cur,ki_cur,umax,ud_form)

persistent up ui temp;

if isempty(up)
    up=0;ui=0;temp=0;
end
ui = ud_form-up;
ui = ui+err*Ts*ki_cur;
up = err*kp_cur;
if(ui>umax)
    ui = umax;
elseif(ui<-umax)
    ui =  -umax;
end
temp = ui+up;
if(temp>umax)
    temp = umax;
elseif(temp<-umax)
    temp =  -umax;
end

iqout = temp;

== matlab function FAN_FW/ASR/speed_PI ==
  data: err input; speedout output; Ts input; kp_asr input; ki_asr input; imax input; Hold input; speed_sat output
function [speedout,speed_sat]  = speed_PI(err,Ts,kp_asr,ki_asr,imax,Hold)

persistent up ui temp temp1 temp2 flag step;

if isempty(up)
    up=0;ui=0;temp=0;temp1=0;flag=0;temp2=0;step=0;
end

% step = 0.0001*10;

if (Hold)
%     temp = temp1;
    up = 0;
    temp = ui+up;
else
    if(temp1 == temp)
        ui = ui+err*Ts*ki_asr;
    end
        up = err*kp_asr;
        temp = ui+up;
end
% if(temp>imax)
%     temp1 = imax;
%     flag = 1;
% elseif(temp<-imax)
%     temp1 =  -imax;
% else
%     temp1 = temp;
% end
% 
% if(temp<(temp1-step))
%    temp = temp1-step;
% elseif(temp>(temp1+step))
%     temp = temp1+step;
% end

if(temp>imax)
    temp1 = imax;
    flag = 1;
elseif(temp<-imax)
    temp1 =  -imax;
else
    temp1 = temp;
end

temp2 = temp1;

speed_sat = flag;
speedout = temp1;

== matlab function FAN_FW/D_ACR/DACR_PI ==
  settings: updateMethod=DISCRETE
  data: err input; idout output; Ts input; kp_cur input; ki_cur input; umax input; ud_form input
function idout  = QACR_PI(err,Ts,kp_cur,ki_cur,umax,ud_form)

persistent up ui temp;

if isempty(up)
    up=0;ui=0;temp=0;
end
ui = ud_form-up;
ui = ui+err*Ts*ki_cur;
up = err*kp_cur;
if(ui>umax)
    ui = umax;
elseif(ui<-umax)
    ui =  -umax;
end
temp = ui+up;
if(temp>umax)
    temp = umax;
elseif(temp<-umax)
    temp =  -umax;
end

idout = temp;
